simulink model "fsm_controller"  (R2025b)
settings: Solver=ode4  StartTime=0.0  StopTime=ctrl_Tstop  FixedStep=ctrl_h  RelTol=1e-3
values from neighbouring files (symbols this model uses):
  ctrl_boundary = 0.01    [build_fsm_controller.m]
  ctrl_eta = 0.1    [build_fsm_controller.m]
  ctrl_G = [1 0.2 0.2 0.1 0.05 0.05]    [build_fsm_controller.m]
  ctrl_K1 = [-0.8 -0.3 -0.4 -0.15 -0.05 -0.05]    [build_fsm_controller.m]
  ctrl_K2 = [-0.8 -0.3 -0.4 -0.15 -0.05 -0.05]    [build_fsm_controller.m]
  wind_p = wind_plant_parameters()    [build_fsm_controller.m]
settings Model: Creator=yuexi  LastModifiedBy=yuexi

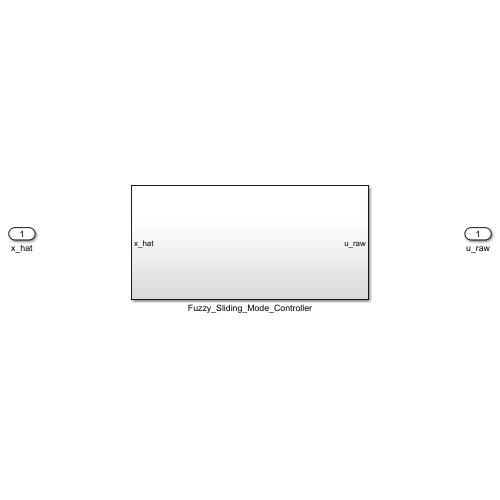
[thumbnail: Simulink's stored preview of the top-level diagram]
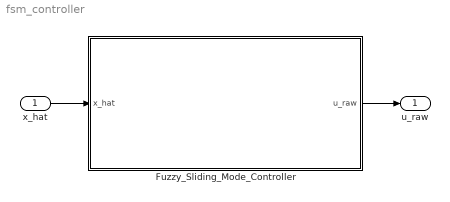
== system fsm_controller ==
  x_hat : Inport
  Fuzzy_Sliding_Mode_Controller : Subsystem
  u_raw : Outport
  wires:
  x_hat/1 -> Fuzzy_Sliding_Mode_Controller/1(x_hat)
  Fuzzy_Sliding_Mode_Controller/1(u_raw) -> u_raw/1

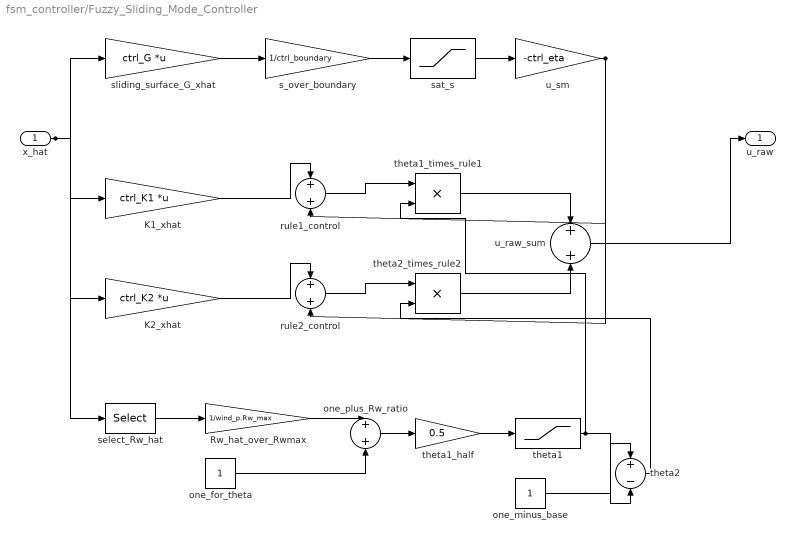
== system fsm_controller/Fuzzy_Sliding_Mode_Controller ==
  x_hat : Inport
  K1_xhat : Gain  Gain=ctrl_K1  Multiplication=Matrix(K*u)
  K2_xhat : Gain  Gain=ctrl_K2  Multiplication=Matrix(K*u)
  Rw_hat_over_Rwmax : Gain  Gain=1/wind_p.Rw_max
  one_for_theta : Constant
  one_minus_base : Constant
  one_plus_Rw_ratio : Sum
  rule1_control : Sum
  rule2_control : Sum
  s_over_boundary : Gain  Gain=1/ctrl_boundary
  sat_s : Saturate  UpperLimit=1  LowerLimit=-1
  select_Rw_hat : Selector  InputPortWidth=6  IndexOptions=Index vector (dialog)  Indices=6  OutputSizes=1
  sliding_surface_G_xhat : Gain  Gain=ctrl_G  Multiplication=Matrix(K*u)
  theta1 : Saturate  UpperLimit=1  LowerLimit=0
  theta1_half : Gain  Gain=0.5
  theta1_times_rule1 : Product
  theta2 : Sum  Inputs=+-
  theta2_times_rule2 : Product
  u_raw_sum : Sum
  u_sm : Gain  Gain=-ctrl_eta
  u_raw : Outport
  wires:
  x_hat/1 -> sliding_surface_G_xhat/1, select_Rw_hat/1, K1_xhat/1, K2_xhat/1
  sliding_surface_G_xhat/1 -> s_over_boundary/1
  s_over_boundary/1 -> sat_s/1
  sat_s/1 -> u_sm/1
  select_Rw_hat/1 -> Rw_hat_over_Rwmax/1
  Rw_hat_over_Rwmax/1 -> one_plus_Rw_ratio/1
  one_for_theta/1 -> one_plus_Rw_ratio/2
  one_plus_Rw_ratio/1 -> theta1_half/1
  theta1_half/1 -> theta1/1
  one_minus_base/1 -> theta2/1
  theta1/1 -> theta2/2, theta1_times_rule1/2
  K1_xhat/1 -> rule1_control/1
  u_sm/1 -> rule1_control/2, rule2_control/2
  K2_xhat/1 -> rule2_control/1
  rule1_control/1 -> theta1_times_rule1/1
  rule2_control/1 -> theta2_times_rule2/1
  theta2/1 -> theta2_times_rule2/2
  theta1_times_rule1/1 -> u_raw_sum/1
  theta2_times_rule2/1 -> u_raw_sum/2
  u_raw_sum/1 -> u_raw/1
